simulink model "simulink7_2_1"  (R2017a)
settings: Solver=VariableStepAuto  StartTime=0.0  StopTime=20.0  RelTol=1e-3
settings Model: Creator=adi  LastModifiedBy=adi

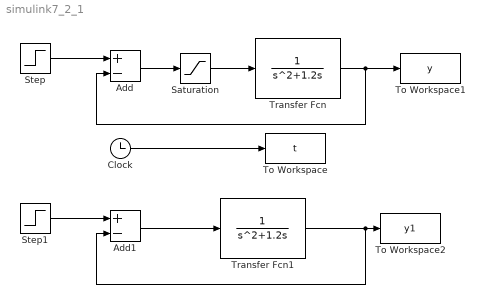
== system simulink7_2_1 ==
  Add : Sum  Inputs=+-
  Add1 : Sum  Inputs=+-
  Clock : Clock
      settings: Decimation=20
  Saturation : Saturate  UpperLimit=0.3  LowerLimit=-0.3
  Step : Step  Time=0  SampleTime=0
  Step1 : Step  Time=0  SampleTime=0
  To Workspace : ToWorkspace  VariableName=t  SampleTime=-1
  To Workspace1 : ToWorkspace  VariableName=y  SampleTime=-1
  To Workspace2 : ToWorkspace  VariableName=y1  SampleTime=-1
  Transfer Fcn : TransferFcn  Denominator=[1 1.2 0]
  Transfer Fcn1 : TransferFcn  Denominator=[1 1.2 0]
  wires:
  Transfer Fcn/1 -> Add/2, To Workspace1/1
  Add/1 -> Saturation/1
  Saturation/1 -> Transfer Fcn/1
  Clock/1 -> To Workspace/1
  Step/1 -> Add/1
  Transfer Fcn1/1 -> Add1/2, To Workspace2/1
  Add1/1 -> Transfer Fcn1/1
  Step1/1 -> Add1/1
